simulink model "param_identified"  (R2016a)
settings: Solver=FixedStepAuto  StartTime=0.0  StopTime=10.0  FixedStep=0.005  RelTol=1e-3
settings Model: Creator=marki  LastModifiedBy=marki

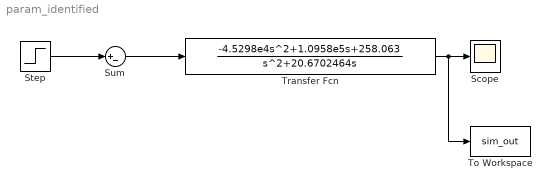
== system param_identified ==
  Scope : Scope
  Step : Step  Time=0  After=8.2786  SampleTime=0
  Sum : Sum  Inputs=|+-
  To Workspace : ToWorkspace  VariableName=sim_out  SaveFormat=Timeseries  SampleTime=-1
  Transfer Fcn : TransferFcn  Numerator=[-4.5298e4 1.0958e5 258.063]  Denominator=[1 20.6702464 0]
  wires:
  Transfer Fcn/1 -> To Workspace/1, Scope/1
  Sum/1 -> Transfer Fcn/1
  Step/1 -> Sum/1
